simulink model "normalization"  (R2023b)
settings: Solver=VariableStepAuto  StartTime=0.0  StopTime=2  RelTol=1e-3
PreLoadFcn:
  | buffer_tiling
InitFcn:
  | buffer_tiling
values from neighbouring files (symbols this model uses):
  COL = 128    [run_model.m]
  inMat1 = reshape(inMat(1:ROW/PLIO_NUM,:)',[],1)    [run_model.m]
  inMat2 = reshape(inMat(ROW/PLIO_NUM+1:ROW/PLIO_NUM*2,:)',[],1)    [run_model.m]
  inMat3 = reshape(inMat(ROW/PLIO_NUM*2+1:ROW,:)',[],1)    [run_model.m]
  ROW = 384    [run_model.m]
undefined symbols (not defined in the file or in its folder): AIE, aie, es1, mean_dev_norm_first, mean_dev_norm_last, mean_dev_norm_middle, ML, mtxA_r, mtxA_w, mtxB_r, mtxB_w, S, vsvh1760, xcve2802
libraries: aieUtilities x14, aieBasic x14, vmcUtilities x1
settings Model: Creator=robg  LastModifiedBy=abehbood
settings DataIOCC: ReturnWorkspaceOutputs=off
settings OptimizationCC: ReuseModelBlockBuffer=off

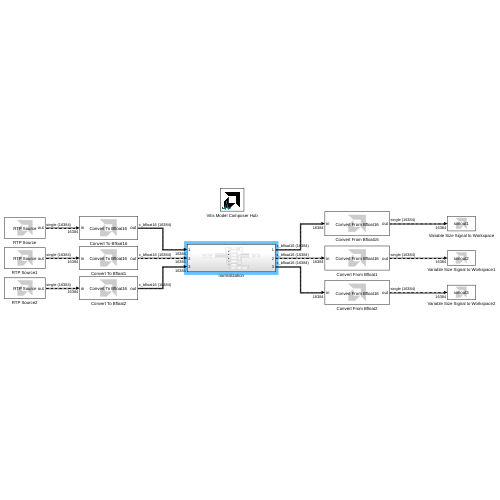
[thumbnail: Simulink's stored preview of the top-level diagram]
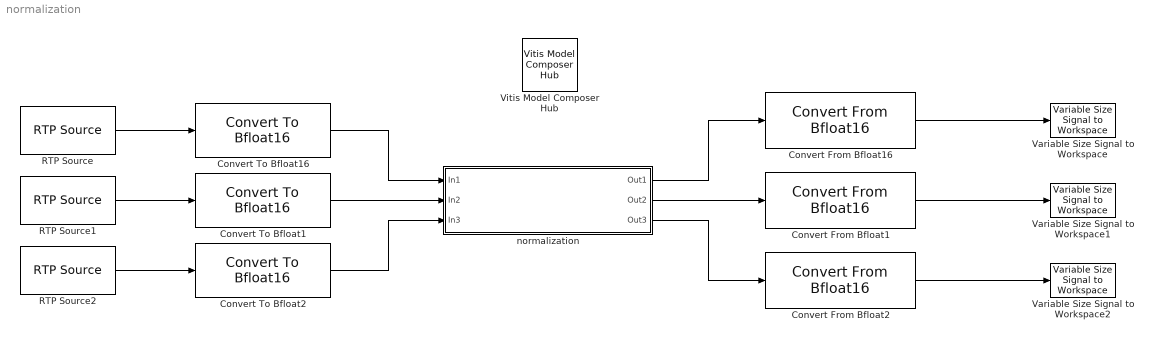
== system normalization ==
  Convert From Bfloat1 : aieUtilities/Convert From Bfloat16  OutputDataType=single
  Convert From Bfloat16 : aieUtilities/Convert From Bfloat16  OutputDataType=single
  Convert From Bfloat2 : aieUtilities/Convert From Bfloat16  OutputDataType=single
  Convert To Bfloat1 : aieUtilities/Convert To Bfloat16
  Convert To Bfloat16 : aieUtilities/Convert To Bfloat16
  Convert To Bfloat2 : aieUtilities/Convert To Bfloat16
  RTP Source : aieUtilities/RTP Source  Value=inMat1  SampleTime=1  OutputForm=Empty
  RTP Source1 : aieUtilities/RTP Source  Value=inMat2  SampleTime=1  OutputForm=Empty
  RTP Source2 : aieUtilities/RTP Source  Value=inMat3  SampleTime=1  OutputForm=Empty
  Variable Size Signal to Workspace : aieUtilities/Variable Size Signal to Workspace  VariableNameMask=simout1
  Variable Size Signal to Workspace1 : aieUtilities/Variable Size Signal to Workspace  VariableNameMask=simout2
  Variable Size Signal to Workspace2 : aieUtilities/Variable Size Signal to Workspace  VariableNameMask=simout3
  Vitis Model Composer Hub : vmcUtilities/Vitis Model Composer Hub  Tag=genX  CodeGeneration=off  SubsystemName=test  CompilationType=AIECompilation  ExportTypeV2=Graph Code  TargetDirectory=./code  exportDesign=off  analyzeDesign=on  validateDesignOnHw=off  ExportType=AI Engines  IpVendor=xilinx.com  IpLibrary=hls  IpVersion=1.0  IpHWLanguage=Verilog  AieCompilerOptions={}  AieSimulatorOptions={}  CreateTestbench=on  TestbenchStackSize=10  RunRtlSim=off  RunCSim=off  RunAieSim=on  AieSimTimeout=50000  RunAieSimProfiling=off  LaunchVitisAnalyzer=off  PlotOutput=off  RunX86Sim=off  X86SimTimeout=10  GenHwImage=off  GenLibadfXo=off  GenHwValidationCode=off  PlatformType=Specify Platform  Platform=/proj/xbuilds/SWIP/9999.0_0214_2115/installs/lin64/Vitis/2024.1/base_platforms/xilinx_vek280_es1_base_202410_1/xilinx_vek280_es1_base_202410_1.xpfm  HwSystemType=Baremetal  HwValidationTarget=hw  ProjDevice=Versal VEK280 ES1 Evaluation Platform with FMC Connector (xcve2802-vsvh1760-2MP-e-S-es1)  ProjDevicePart=xcve2802-vsvh1760-2MP-e-S-es1  AIEType=AIE-ML  SamplePeriod=-1  ClockFrequency=200  DataPathParallelism=1  xilinxfamily=versalaiedgees1  part=xcve2802  speed=-2MP-e-S-es1  package=vsvh1760  directory=./netlist  testbench=off  incr_netlist=off  synthesis_tool=Vivado  clock_wrapper=Clock Enables  dbl_ovrd=According to Block Masks  dcm_input_clock_period=10  sysclk_period=10  simulink_period=1  eval_field=0  IPInfoJsonString="{\"AIESubsystem\":{\"SubsystemName\":\"test\",\"TargetDirectory\":\"./code\",\"SubsystemDir\":\"./code/ip/test\"},\"SubsystemTag\":\"AIENode\"}"  LogFileName=/proj/xsjhdstaff4/abehbood/customers/AIE-ML_Performance_Analysis/normalization_v4/code/model_composer.log  NThreads=4
  normalization : Subsystem
  wires:
  RTP Source/1 -> Convert To Bfloat16/1
  Convert To Bfloat16/1 -> normalization/1(In1)
  normalization/1(Out1) -> Convert From Bfloat16/1
  Convert To Bfloat1/1 -> normalization/2(In2)
  RTP Source1/1 -> Convert To Bfloat1/1
  Convert To Bfloat2/1 -> normalization/3(In3)
  RTP Source2/1 -> Convert To Bfloat2/1
  normalization/2(Out2) -> Convert From Bfloat1/1
  normalization/3(Out3) -> Convert From Bfloat2/1
  Convert From Bfloat16/1 -> Variable Size Signal to Workspace/1
  Convert From Bfloat1/1 -> Variable Size Signal to Workspace1/1
  Convert From Bfloat2/1 -> Variable Size Signal to Workspace2/1

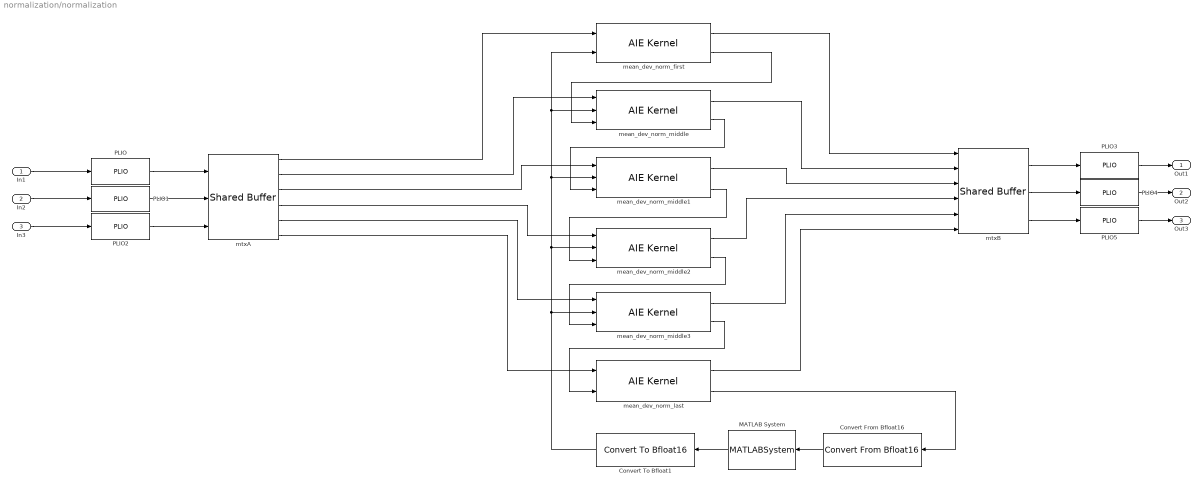
== system normalization/normalization ==
  In1 : Inport
  In2 : Inport  Port=2
  In3 : Inport  Port=3
  Convert From Bfloat16 : aieUtilities/Convert From Bfloat16  OutputDataType=single
  Convert To Bfloat1 : aieUtilities/Convert To Bfloat16
  MATLAB System : MATLABSystem  System=cycleBreaker  SimulateUsing=Interpreted execution
      mask Type: cycleBreaker
      mask Display:
      | disp('cycleBreaker');
      | port_label('input',1,'u');
      | port_label('output',1,'y');
  PLIO{,1..5} (6 alike) : aieBasic/PLIO  PlioWidth=128  PlioFreqSpec=off  PlioFreq=250  ColLocation=0  channel=0  blockJsonConstraints=[]  deprecateConstraints=0
  mean_dev_norm_first : aieBasic/AIE Kernel  KernelAllAttrs=|  PortNames={'data'; 'mean_dev'; 'out'; 'partial_out'}  PortSerializedTypes={'{Q2{R{Tadf::input_buffer{1{t{Sbfloat16}}}}}}'; '{Q2{P{Tinput_stream{1{t{Sbfloat16}}}}}}'; '{Q2{R{Tadf::output_buffer{1{t{Sbfloat16}}}}}}'; '{Q2{P{Toutput_cascade{2{t{Saccfloat}}{t{Bv}}}}}}'}  PortWindowSizes={8.192000000000000000e+03, 0.000000000000000000e+00, 8.192000000000000000e+03, 0.000000000000000000e+00}  PortWindowMargins={0.000000000000000000e+00, 0.000000000000000000e+00, 0.000000000000000000e+00, 0.000000000000000000e+00}  PortSynchronicities={'sync', 'auto', 'sync', 'auto'}  PortSignalSizes={0.000000000000000000e+00; 0.000000000000000000e+00; 0.000000000000000000e+00; 3.200000000000000000e+01}  FunctionTemplateSpecKind=implicit  FunctionTemplateParamNames={'COL'; 'ROW'}  FunctionTemplateParamKinds={'nontype'; 'nontype'}  FunctionTemplateParamTypes={'int'; 'int'}  FunctionTemplateParamValues={'128', '64'}  FunctionIndex=1  FunctionTabVisible=on  FunctionTemplateParamsVisible=on  FunctionDeclTypeOptions=|  FunctionDecl=|  FunctionTemplateParams={ 'COL', 'int', 'K_COL'; 'ROW', 'int', 'K_ROW' }  FunctionTemplateParamsEnables={'off', 'off', 'on';'off', 'off', 'on'}  PortAttrs={ 'input', 'data', 'adf::input_buffer< bfloat16 > & restrict', 'K_COL*K_ROW', '0', 'sync', ''; 'input', 'mean_dev', 'input_stream< bfloat16 > * restrict', '', '', '', ''; 'output', 'out', 'adf::output_buffer< bfloat16 > & restrict', 'K_COL*K_ROW', '', 'sync', ''; 'output', 'partial_out', 'output_cascade< accfloat, void > * restrict', '', '', '', '32' }  PortAttrsEnables={'off', 'off', 'off', 'on', 'off', 'off', 'off';'off', 'off', 'off', 'off', 'off', 'off', 'off';'off', 'off', 'off', 'on', 'off', 'off', 'off';'off', 'off', 'off', 'off', 'off', 'off', 'on'}  SampleTime=-1  KernelHeaderFile=aie/kernels.h  KernelFunction=mean_dev_norm_first  KernelSourceFile=aie/mean_dev_norm_first.cc  KernelSearchPaths={}  PreProcOptions={}  blockJsonConstraints=[]
      KernelAllAttrs=|
      | s[12;12;9;9;19;14;21;23;21;23;24;21;15;17;12;24;26;26;26;27;28;9;21;23;23;23;24;25;14;19;19;29]@FunctionNameDeclFileNamePortNamesPortTypesPortSerializedTypesPortDirectionsPortWindowSizeEnablesPortWindowMarginEnablesPortBufferSizeEnablesPortBufferMarginEnablesPortSynchronicityEnablesPortSignalSizeEnablesPortBufferSizesPortBufferMarginsFunctionDeclFunctionTemplateSpecKindFunctionTemplateParamNamesFunctionTemplateParamKindsFunctionTemplateParamTypesFunctionTemplateParamValuesFunctionTemplateParamEnablesClassDeclClassTemplateSpecKindClassTemplateParamNamesClassTemplateParamKindsClassTemplateParamTypesClassTemplateParamValuesClassTemplateParamEnablesClassCtorDeclsClassCtorParamNamesClassCtorParamTypesClassCtorParamSerializedTypes[1 1]@C[32 1]@t19@mean_dev_norm_firstt19@../../aie/kernels.hC[4 1]@t4@datat8@mean_devt3@outt11@partial_outC[4 1]@t40@adf::input_buffer< bfloat16 > & restrictt35@input_stream< bfloat16 > * restrictt41@adf::output_buffer< bfloat16 > & restrictt43@output_cascade< accfloat, void > * restrictC[4 1]@t44@{Q2{R{Tadf::input_buffer{1{t{Sbfloat16}}}}}}t39@{Q2{P{Tinput_stream{1{t{Sbfloat16}}}}}}t45@{Q2{R{Tadf::output_buffer{1{t{Sbfloat16}}}}}}t48@{Q2{P{Toutput_cascade{2{t{Saccfloat}}{t{Bv}}}}}}C[4 1]@t5@inputt5@inputt6@outputt6@outputC[4 1]@l1@l0@l1@l0@C[4 1]@l1@l0@l0@l0@C[4 1]@l1@l0@l1@l0@C[4 1]@l0@l0@l0@l0@C[4 1]@l1@l0@l1@l0@C[4 1]@l0@l0@l0@l1@C[4 1]@nnnnC[4 1]@nnnnt252@template < int COL, int ROW > 
      | void mean_dev_norm_first(adf::input_buffer< bfloat16 > & restrict data, input_stream< bfloat16 > * restrict mean_dev, adf::output_buffer< bfloat16 > & restrict out, output_cascade< accfloat, void > * restrict partial_out)t8@implicitC[2 1]@t3@COLt3@ROWC[2 1]@t7@nontypet7@nontypeC[2 1]@t3@intt3@intC[2 1]@nnC[2 1]@l1@l1@nne[0 1]@e[0 1]@e[0 1]@e[0 1]@e[0 1]@e[0 1]@e[0 1]@e[0 1]@e[0 1]@
      FunctionDeclTypeOptions=|
      | C[1 1]@t254@template < int COL, int ROW > 
      | void mean_dev_norm_first(adf::input_buffer< bfloat16 > && restrict data, input_stream< bfloat16 > * restrict mean_dev, adf::output_buffer< bfloat16 > && restrict out, output_cascade< accfloat, void > * restrict partial_out)
      FunctionDecl=|
      | template < int COL, int ROW > 
      | void mean_dev_norm_first(adf::input_buffer< bfloat16 > && restrict data, input_stream< bfloat16 > * restrict mean_dev, adf::output_buffer< bfloat16 > && restrict out, output_cascade< accfloat, void > * restrict partial_out)
  mean_dev_norm_last : aieBasic/AIE Kernel  KernelAllAttrs=|  PortNames={'data'; 'partial_in'; 'out'; 'mean_dev_out'}  PortSerializedTypes={'{Q2{R{Tadf::input_buffer{1{t{Sbfloat16}}}}}}'; '{Q2{P{Tinput_cascade{2{t{Saccfloat}}{t{Bv}}}}}}'; '{Q2{R{Tadf::output_buffer{1{t{Sbfloat16}}}}}}'; '{Q2{P{Toutput_stream{1{t{Sbfloat16}}}}}}'}  PortWindowSizes={8.192000000000000000e+03, 0.000000000000000000e+00, 8.192000000000000000e+03, 0.000000000000000000e+00}  PortWindowMargins={0.000000000000000000e+00, 0.000000000000000000e+00, 0.000000000000000000e+00, 0.000000000000000000e+00}  PortSynchronicities={'sync', 'auto', 'sync', 'auto'}  PortSignalSizes={0.000000000000000000e+00; 0.000000000000000000e+00; 0.000000000000000000e+00; 2.000000000000000000e+00}  FunctionTemplateSpecKind=implicit  FunctionTemplateParamNames={'COL'; 'ROW'; 'NUM'}  FunctionTemplateParamKinds={'nontype'; 'nontype'; 'nontype'}  FunctionTemplateParamTypes={'int'; 'int'; 'int'}  FunctionTemplateParamValues={'128', '64', '6'}  FunctionIndex=1  FunctionTabVisible=on  FunctionTemplateParamsVisible=on  FunctionDeclTypeOptions=|  FunctionDecl=|  FunctionTemplateParams={ 'COL', 'int', 'K_COL'; 'ROW', 'int', 'K_ROW'; 'NUM', 'int', 'NUM' }  FunctionTemplateParamsEnables={'off', 'off', 'on';'off', 'off', 'on';'off', 'off', 'on'}  PortAttrs={ 'input', 'data', 'adf::input_buffer< bfloat16 > & restrict', 'K_COL*K_ROW', '0', 'sync', ''; 'input', 'partial_in', 'input_cascade< accfloat, void > * restrict', '', '', '', ''; 'output', 'out', 'adf::output_buffer< bfloat16 > & restrict', 'K_COL*K_ROW', '', 'sync', ''; 'output', 'mean_dev_out', 'output_stream< bfloat16 > * restrict', '', '', '', '2' }  PortAttrsEnables={'off', 'off', 'off', 'on', 'off', 'off', 'off';'off', 'off', 'off', 'off', 'off', 'off', 'off';'off', 'off', 'off', 'on', 'off', 'off', 'off';'off', 'off', 'off', 'off', 'off', 'off', 'on'}  SampleTime=-1  KernelHeaderFile=aie/kernels.h  KernelFunction=mean_dev_norm_last  KernelSourceFile=aie/mean_dev_norm_last.cc  KernelSearchPaths={}  PreProcOptions={}  blockJsonConstraints=[]
      KernelAllAttrs=|
      | s[12;12;9;9;19;14;21;23;21;23;24;21;15;17;12;24;26;26;26;27;28;9;21;23;23;23;24;25;14;19;19;29]@FunctionNameDeclFileNamePortNamesPortTypesPortSerializedTypesPortDirectionsPortWindowSizeEnablesPortWindowMarginEnablesPortBufferSizeEnablesPortBufferMarginEnablesPortSynchronicityEnablesPortSignalSizeEnablesPortBufferSizesPortBufferMarginsFunctionDeclFunctionTemplateSpecKindFunctionTemplateParamNamesFunctionTemplateParamKindsFunctionTemplateParamTypesFunctionTemplateParamValuesFunctionTemplateParamEnablesClassDeclClassTemplateSpecKindClassTemplateParamNamesClassTemplateParamKindsClassTemplateParamTypesClassTemplateParamValuesClassTemplateParamEnablesClassCtorDeclsClassCtorParamNamesClassCtorParamTypesClassCtorParamSerializedTypes[1 1]@C[32 1]@t18@mean_dev_norm_lastt19@../../aie/kernels.hC[4 1]@t4@datat10@partial_int3@outt12@mean_dev_outC[4 1]@t40@adf::input_buffer< bfloat16 > & restrictt42@input_cascade< accfloat, void > * restrictt41@adf::output_buffer< bfloat16 > & restrictt36@output_stream< bfloat16 > * restrictC[4 1]@t44@{Q2{R{Tadf::input_buffer{1{t{Sbfloat16}}}}}}t47@{Q2{P{Tinput_cascade{2{t{Saccfloat}}{t{Bv}}}}}}t45@{Q2{R{Tadf::output_buffer{1{t{Sbfloat16}}}}}}t40@{Q2{P{Toutput_stream{1{t{Sbfloat16}}}}}}C[4 1]@t5@inputt5@inputt6@outputt6@outputC[4 1]@l1@l0@l1@l0@C[4 1]@l1@l0@l0@l0@C[4 1]@l1@l0@l1@l0@C[4 1]@l0@l0@l0@l0@C[4 1]@l1@l0@l1@l0@C[4 1]@l0@l0@l0@l1@C[4 1]@nnnnC[4 1]@nnnnt263@template < int COL, int ROW, int NUM > 
      | void mean_dev_norm_last(adf::input_buffer< bfloat16 > & restrict data, input_cascade< accfloat, void > * restrict partial_in, adf::output_buffer< bfloat16 > & restrict out, output_stream< bfloat16 > * restrict mean_dev_out)t8@implicitC[3 1]@t3@COLt3@ROWt3@NUMC[3 1]@t7@nontypet7@nontypet7@nontypeC[3 1]@t3@intt3@intt3@intC[3 1]@nnnC[3 1]@l1@l1@l1@nne[0 1]@e[0 1]@e[0 1]@e[0 1]@e[0 1]@e[0 1]@e[0 1]@e[0 1]@e[0 1]@
      FunctionDeclTypeOptions=|
      | C[1 1]@t265@template < int COL, int ROW, int NUM > 
      | void mean_dev_norm_last(adf::input_buffer< bfloat16 > && restrict data, input_cascade< accfloat, void > * restrict partial_in, adf::output_buffer< bfloat16 > && restrict out, output_stream< bfloat16 > * restrict mean_dev_out)
      FunctionDecl=|
      | template < int COL, int ROW, int NUM > 
      | void mean_dev_norm_last(adf::input_buffer< bfloat16 > && restrict data, input_cascade< accfloat, void > * restrict partial_in, adf::output_buffer< bfloat16 > && restrict out, output_stream< bfloat16 > * restrict mean_dev_out)
  mean_dev_norm_middle : aieBasic/AIE Kernel  KernelAllAttrs=|  PortNames={'data'; 'mean_dev'; 'partial_in'; 'out'; 'partial_out'}  PortSerializedTypes={'{Q2{R{Tadf::input_buffer{1{t{Sbfloat16}}}}}}'; '{Q2{P{Tinput_stream{1{t{Sbfloat16}}}}}}'; '{Q2{P{Tinput_cascade{2{t{Saccfloat}}{t{Bv}}}}}}'; '{Q2{R{Tadf::output_buffer{1{t{Sbfloat16}}}}}}'; '{Q2{P{Toutput_cascade{2{t{Saccfloat}}{t{Bv}}}}}}'}  PortWindowSizes={8.192000000000000000e+03, 0.000000000000000000e+00, 0.000000000000000000e+00, 8.192000000000000000e+03, 0.000000000000000000e+00}  PortWindowMargins={0.000000000000000000e+00, 0.000000000000000000e+00, 0.000000000000000000e+00, 0.000000000000000000e+00, 0.000000000000000000e+00}  PortSynchronicities={'sync', 'auto', 'auto', 'sync', 'auto'}  PortSignalSizes={0.000000000000000000e+00; 0.000000000000000000e+00; 0.000000000000000000e+00; 0.000000000000000000e+00; 3.200000000000000000e+01}  FunctionTemplateSpecKind=implicit  FunctionTemplateParamNames={'COL'; 'ROW'}  FunctionTemplateParamKinds={'nontype'; 'nontype'}  FunctionTemplateParamTypes={'int'; 'int'}  FunctionTemplateParamValues={'128', '64'}  FunctionIndex=1  FunctionTabVisible=on  FunctionTemplateParamsVisible=on  FunctionDeclTypeOptions=|  FunctionDecl=|  FunctionTemplateParams={ 'COL', 'int', 'K_COL'; 'ROW', 'int', 'K_ROW' }  FunctionTemplateParamsEnables={'off', 'off', 'on';'off', 'off', 'on'}  PortAttrs={ 'input', 'data', 'adf::input_buffer< bfloat16 > & restrict', 'K_COL*K_ROW', '0', 'sync', ''; 'input', 'mean_dev', 'input_stream< bfloat16 > * restrict', '', '', '', ''; 'input', 'partial_in', 'input_cascade< accfloat, void > * restrict', '', '', '', ''; 'output', 'out', 'adf::output_buffer< bfloat16 > & restrict', 'K_COL*K_ROW', '', 'sync', ''; 'output', 'partial_out', 'output_cascade< accfloat, void > * restrict', '', '', '', '32' }  PortAttrsEnables={'off', 'off', 'off', 'on', 'off', 'off', 'off';'off', 'off', 'off', 'off', 'off', 'off', 'off';'off', 'off', 'off', 'off', 'off', 'off', 'off';'off', 'off', 'off', 'on', 'off', 'off', 'off';'off', 'off', 'off', 'off', 'off', 'off', 'on'}  SampleTime=-1  KernelHeaderFile=aie/kernels.h  KernelFunction=mean_dev_norm_middle  KernelSourceFile=aie/mean_dev_norm_middle.cc  KernelSearchPaths={}  PreProcOptions={}  blockJsonConstraints=[]
      KernelAllAttrs=|
      | s[12;12;9;9;19;14;21;23;21;23;24;21;15;17;12;24;26;26;26;27;28;9;21;23;23;23;24;25;14;19;19;29]@FunctionNameDeclFileNamePortNamesPortTypesPortSerializedTypesPortDirectionsPortWindowSizeEnablesPortWindowMarginEnablesPortBufferSizeEnablesPortBufferMarginEnablesPortSynchronicityEnablesPortSignalSizeEnablesPortBufferSizesPortBufferMarginsFunctionDeclFunctionTemplateSpecKindFunctionTemplateParamNamesFunctionTemplateParamKindsFunctionTemplateParamTypesFunctionTemplateParamValuesFunctionTemplateParamEnablesClassDeclClassTemplateSpecKindClassTemplateParamNamesClassTemplateParamKindsClassTemplateParamTypesClassTemplateParamValuesClassTemplateParamEnablesClassCtorDeclsClassCtorParamNamesClassCtorParamTypesClassCtorParamSerializedTypes[1 1]@C[32 1]@t20@mean_dev_norm_middlet19@../../aie/kernels.hC[5 1]@t4@datat8@mean_devt10@partial_int3@outt11@partial_outC[5 1]@t40@adf::input_buffer< bfloat16 > & restrictt35@input_stream< bfloat16 > * restrictt42@input_cascade< accfloat, void > * restrictt41@adf::output_buffer< bfloat16 > & restrictt43@output_cascade< accfloat, void > * restrictC[5 1]@t44@{Q2{R{Tadf::input_buffer{1{t{Sbfloat16}}}}}}t39@{Q2{P{Tinput_stream{1{t{Sbfloat16}}}}}}t47@{Q2{P{Tinput_cascade{2{t{Saccfloat}}{t{Bv}}}}}}t45@{Q2{R{Tadf::output_buffer{1{t{Sbfloat16}}}}}}t48@{Q2{P{Toutput_cascade{2{t{Saccfloat}}{t{Bv}}}}}}C[5 1]@t5@inputt5@inputt5@inputt6@outputt6@outputC[5 1]@l1@l0@l0@l1@l0@C[5 1]@l1@l0@l0@l0@l0@C[5 1]@l1@l0@l0@l1@l0@C[5 1]@l0@l0@l0@l0@l0@C[5 1]@l1@l0@l0@l1@l0@C[5 1]@l0@l0@l0@l0@l1@C[5 1]@nnnnnC[5 1]@nnnnnt308@template < int COL, int ROW > 
      | void mean_dev_norm_middle(adf::input_buffer< bfloat16 > & restrict data, input_stream< bfloat16 > * restrict mean_dev, input_cascade< accfloat, void > * restrict partial_in, adf::output_buffer< bfloat16 > & restrict out, output_cascade< accfloat, void > * restrict partial_out)t8@implicitC[2 1]@t3@COLt3@ROWC[2 1]@t7@nontypet7@nontypeC[2 1]@t3@intt3@intC[2 1]@nnC[2 1]@l1@l1@nne[0 1]@e[0 1]@e[0 1]@e[0 1]@e[0 1]@e[0 1]@e[0 1]@e[0 1]@e[0 1]@
      FunctionDeclTypeOptions=|
      | C[1 1]@t310@template < int COL, int ROW > 
      | void mean_dev_norm_middle(adf::input_buffer< bfloat16 > && restrict data, input_stream< bfloat16 > * restrict mean_dev, input_cascade< accfloat, void > * restrict partial_in, adf::output_buffer< bfloat16 > && restrict out, output_cascade< accfloat, void > * restrict partial_out)
      FunctionDecl=|
      | template < int COL, int ROW > 
      | void mean_dev_norm_middle(adf::input_buffer< bfloat16 > && restrict data, input_stream< bfloat16 > * restrict mean_dev, input_cascade< accfloat, void > * restrict partial_in, adf::output_buffer< bfloat16 > && restrict out, output_cascade< accfloat, void > * restrict partial_out)
  mean_dev_norm_middle1 : aieBasic/AIE Kernel  KernelAllAttrs=|  PortNames={'data'; 'mean_dev'; 'partial_in'; 'out'; 'partial_out'}  PortSerializedTypes={'{Q2{R{Tadf::input_buffer{1{t{Sbfloat16}}}}}}'; '{Q2{P{Tinput_stream{1{t{Sbfloat16}}}}}}'; '{Q2{P{Tinput_cascade{2{t{Saccfloat}}{t{Bv}}}}}}'; '{Q2{R{Tadf::output_buffer{1{t{Sbfloat16}}}}}}'; '{Q2{P{Toutput_cascade{2{t{Saccfloat}}{t{Bv}}}}}}'}  PortWindowSizes={8.192000000000000000e+03, 0.000000000000000000e+00, 0.000000000000000000e+00, 8.192000000000000000e+03, 0.000000000000000000e+00}  PortWindowMargins={0.000000000000000000e+00, 0.000000000000000000e+00, 0.000000000000000000e+00, 0.000000000000000000e+00, 0.000000000000000000e+00}  PortSynchronicities={'sync', 'auto', 'auto', 'sync', 'auto'}  PortSignalSizes={0.000000000000000000e+00; 0.000000000000000000e+00; 0.000000000000000000e+00; 0.000000000000000000e+00; 3.200000000000000000e+01}  FunctionTemplateSpecKind=implicit  FunctionTemplateParamNames={'COL'; 'ROW'}  FunctionTemplateParamKinds={'nontype'; 'nontype'}  FunctionTemplateParamTypes={'int'; 'int'}  FunctionTemplateParamValues={'128', '64'}  FunctionIndex=1  FunctionTabVisible=on  FunctionTemplateParamsVisible=on  FunctionDeclTypeOptions=|  FunctionDecl=|  FunctionTemplateParams={ 'COL', 'int', 'K_COL'; 'ROW', 'int', 'K_ROW' }  FunctionTemplateParamsEnables={'off', 'off', 'on';'off', 'off', 'on'}  PortAttrs={ 'input', 'data', 'adf::input_buffer< bfloat16 > & restrict', 'K_COL*K_ROW', '0', 'sync', ''; 'input', 'mean_dev', 'input_stream< bfloat16 > * restrict', '', '', '', ''; 'input', 'partial_in', 'input_cascade< accfloat, void > * restrict', '', '', '', ''; 'output', 'out', 'adf::output_buffer< bfloat16 > & restrict', 'K_COL*K_ROW', '', 'sync', ''; 'output', 'partial_out', 'output_cascade< accfloat, void > * restrict', '', '', '', '32' }  PortAttrsEnables={'off', 'off', 'off', 'on', 'off', 'off', 'off';'off', 'off', 'off', 'off', 'off', 'off', 'off';'off', 'off', 'off', 'off', 'off', 'off', 'off';'off', 'off', 'off', 'on', 'off', 'off', 'off';'off', 'off', 'off', 'off', 'off', 'off', 'on'}  SampleTime=-1  KernelHeaderFile=aie/kernels.h  KernelFunction=mean_dev_norm_middle  KernelSourceFile=aie/mean_dev_norm_middle.cc  KernelSearchPaths={}  PreProcOptions={}  blockJsonConstraints=[]
      KernelAllAttrs=|
      | s[12;12;9;9;19;14;21;23;21;23;24;21;15;17;12;24;26;26;26;27;28;9;21;23;23;23;24;25;14;19;19;29]@FunctionNameDeclFileNamePortNamesPortTypesPortSerializedTypesPortDirectionsPortWindowSizeEnablesPortWindowMarginEnablesPortBufferSizeEnablesPortBufferMarginEnablesPortSynchronicityEnablesPortSignalSizeEnablesPortBufferSizesPortBufferMarginsFunctionDeclFunctionTemplateSpecKindFunctionTemplateParamNamesFunctionTemplateParamKindsFunctionTemplateParamTypesFunctionTemplateParamValuesFunctionTemplateParamEnablesClassDeclClassTemplateSpecKindClassTemplateParamNamesClassTemplateParamKindsClassTemplateParamTypesClassTemplateParamValuesClassTemplateParamEnablesClassCtorDeclsClassCtorParamNamesClassCtorParamTypesClassCtorParamSerializedTypes[1 1]@C[32 1]@t20@mean_dev_norm_middlet19@../../aie/kernels.hC[5 1]@t4@datat8@mean_devt10@partial_int3@outt11@partial_outC[5 1]@t40@adf::input_buffer< bfloat16 > & restrictt35@input_stream< bfloat16 > * restrictt42@input_cascade< accfloat, void > * restrictt41@adf::output_buffer< bfloat16 > & restrictt43@output_cascade< accfloat, void > * restrictC[5 1]@t44@{Q2{R{Tadf::input_buffer{1{t{Sbfloat16}}}}}}t39@{Q2{P{Tinput_stream{1{t{Sbfloat16}}}}}}t47@{Q2{P{Tinput_cascade{2{t{Saccfloat}}{t{Bv}}}}}}t45@{Q2{R{Tadf::output_buffer{1{t{Sbfloat16}}}}}}t48@{Q2{P{Toutput_cascade{2{t{Saccfloat}}{t{Bv}}}}}}C[5 1]@t5@inputt5@inputt5@inputt6@outputt6@outputC[5 1]@l1@l0@l0@l1@l0@C[5 1]@l1@l0@l0@l0@l0@C[5 1]@l1@l0@l0@l1@l0@C[5 1]@l0@l0@l0@l0@l0@C[5 1]@l1@l0@l0@l1@l0@C[5 1]@l0@l0@l0@l0@l1@C[5 1]@nnnnnC[5 1]@nnnnnt308@template < int COL, int ROW > 
      | void mean_dev_norm_middle(adf::input_buffer< bfloat16 > & restrict data, input_stream< bfloat16 > * restrict mean_dev, input_cascade< accfloat, void > * restrict partial_in, adf::output_buffer< bfloat16 > & restrict out, output_cascade< accfloat, void > * restrict partial_out)t8@implicitC[2 1]@t3@COLt3@ROWC[2 1]@t7@nontypet7@nontypeC[2 1]@t3@intt3@intC[2 1]@nnC[2 1]@l1@l1@nne[0 1]@e[0 1]@e[0 1]@e[0 1]@e[0 1]@e[0 1]@e[0 1]@e[0 1]@e[0 1]@
      FunctionDeclTypeOptions=|
      | C[1 1]@t310@template < int COL, int ROW > 
      | void mean_dev_norm_middle(adf::input_buffer< bfloat16 > && restrict data, input_stream< bfloat16 > * restrict mean_dev, input_cascade< accfloat, void > * restrict partial_in, adf::output_buffer< bfloat16 > && restrict out, output_cascade< accfloat, void > * restrict partial_out)
      FunctionDecl=|
      | template < int COL, int ROW > 
      | void mean_dev_norm_middle(adf::input_buffer< bfloat16 > && restrict data, input_stream< bfloat16 > * restrict mean_dev, input_cascade< accfloat, void > * restrict partial_in, adf::output_buffer< bfloat16 > && restrict out, output_cascade< accfloat, void > * restrict partial_out)
  mean_dev_norm_middle2 : aieBasic/AIE Kernel  KernelAllAttrs=|  PortNames={'data'; 'mean_dev'; 'partial_in'; 'out'; 'partial_out'}  PortSerializedTypes={'{Q2{R{Tadf::input_buffer{1{t{Sbfloat16}}}}}}'; '{Q2{P{Tinput_stream{1{t{Sbfloat16}}}}}}'; '{Q2{P{Tinput_cascade{2{t{Saccfloat}}{t{Bv}}}}}}'; '{Q2{R{Tadf::output_buffer{1{t{Sbfloat16}}}}}}'; '{Q2{P{Toutput_cascade{2{t{Saccfloat}}{t{Bv}}}}}}'}  PortWindowSizes={8.192000000000000000e+03, 0.000000000000000000e+00, 0.000000000000000000e+00, 8.192000000000000000e+03, 0.000000000000000000e+00}  PortWindowMargins={0.000000000000000000e+00, 0.000000000000000000e+00, 0.000000000000000000e+00, 0.000000000000000000e+00, 0.000000000000000000e+00}  PortSynchronicities={'sync', 'auto', 'auto', 'sync', 'auto'}  PortSignalSizes={0.000000000000000000e+00; 0.000000000000000000e+00; 0.000000000000000000e+00; 0.000000000000000000e+00; 3.200000000000000000e+01}  FunctionTemplateSpecKind=implicit  FunctionTemplateParamNames={'COL'; 'ROW'}  FunctionTemplateParamKinds={'nontype'; 'nontype'}  FunctionTemplateParamTypes={'int'; 'int'}  FunctionTemplateParamValues={'128', '64'}  FunctionIndex=1  FunctionTabVisible=on  FunctionTemplateParamsVisible=on  FunctionDeclTypeOptions=|  FunctionDecl=|  FunctionTemplateParams={ 'COL', 'int', 'K_COL'; 'ROW', 'int', 'K_ROW' }  FunctionTemplateParamsEnables={'off', 'off', 'on';'off', 'off', 'on'}  PortAttrs={ 'input', 'data', 'adf::input_buffer< bfloat16 > & restrict', 'K_COL*K_ROW', '0', 'sync', ''; 'input', 'mean_dev', 'input_stream< bfloat16 > * restrict', '', '', '', ''; 'input', 'partial_in', 'input_cascade< accfloat, void > * restrict', '', '', '', ''; 'output', 'out', 'adf::output_buffer< bfloat16 > & restrict', 'K_COL*K_ROW', '', 'sync', ''; 'output', 'partial_out', 'output_cascade< accfloat, void > * restrict', '', '', '', '32' }  PortAttrsEnables={'off', 'off', 'off', 'on', 'off', 'off', 'off';'off', 'off', 'off', 'off', 'off', 'off', 'off';'off', 'off', 'off', 'off', 'off', 'off', 'off';'off', 'off', 'off', 'on', 'off', 'off', 'off';'off', 'off', 'off', 'off', 'off', 'off', 'on'}  SampleTime=-1  KernelHeaderFile=aie/kernels.h  KernelFunction=mean_dev_norm_middle  KernelSourceFile=aie/mean_dev_norm_middle.cc  KernelSearchPaths={}  PreProcOptions={}  blockJsonConstraints=[]
      KernelAllAttrs=|
      | s[12;12;9;9;19;14;21;23;21;23;24;21;15;17;12;24;26;26;26;27;28;9;21;23;23;23;24;25;14;19;19;29]@FunctionNameDeclFileNamePortNamesPortTypesPortSerializedTypesPortDirectionsPortWindowSizeEnablesPortWindowMarginEnablesPortBufferSizeEnablesPortBufferMarginEnablesPortSynchronicityEnablesPortSignalSizeEnablesPortBufferSizesPortBufferMarginsFunctionDeclFunctionTemplateSpecKindFunctionTemplateParamNamesFunctionTemplateParamKindsFunctionTemplateParamTypesFunctionTemplateParamValuesFunctionTemplateParamEnablesClassDeclClassTemplateSpecKindClassTemplateParamNamesClassTemplateParamKindsClassTemplateParamTypesClassTemplateParamValuesClassTemplateParamEnablesClassCtorDeclsClassCtorParamNamesClassCtorParamTypesClassCtorParamSerializedTypes[1 1]@C[32 1]@t20@mean_dev_norm_middlet19@../../aie/kernels.hC[5 1]@t4@datat8@mean_devt10@partial_int3@outt11@partial_outC[5 1]@t40@adf::input_buffer< bfloat16 > & restrictt35@input_stream< bfloat16 > * restrictt42@input_cascade< accfloat, void > * restrictt41@adf::output_buffer< bfloat16 > & restrictt43@output_cascade< accfloat, void > * restrictC[5 1]@t44@{Q2{R{Tadf::input_buffer{1{t{Sbfloat16}}}}}}t39@{Q2{P{Tinput_stream{1{t{Sbfloat16}}}}}}t47@{Q2{P{Tinput_cascade{2{t{Saccfloat}}{t{Bv}}}}}}t45@{Q2{R{Tadf::output_buffer{1{t{Sbfloat16}}}}}}t48@{Q2{P{Toutput_cascade{2{t{Saccfloat}}{t{Bv}}}}}}C[5 1]@t5@inputt5@inputt5@inputt6@outputt6@outputC[5 1]@l1@l0@l0@l1@l0@C[5 1]@l1@l0@l0@l0@l0@C[5 1]@l1@l0@l0@l1@l0@C[5 1]@l0@l0@l0@l0@l0@C[5 1]@l1@l0@l0@l1@l0@C[5 1]@l0@l0@l0@l0@l1@C[5 1]@nnnnnC[5 1]@nnnnnt308@template < int COL, int ROW > 
      | void mean_dev_norm_middle(adf::input_buffer< bfloat16 > & restrict data, input_stream< bfloat16 > * restrict mean_dev, input_cascade< accfloat, void > * restrict partial_in, adf::output_buffer< bfloat16 > & restrict out, output_cascade< accfloat, void > * restrict partial_out)t8@implicitC[2 1]@t3@COLt3@ROWC[2 1]@t7@nontypet7@nontypeC[2 1]@t3@intt3@intC[2 1]@nnC[2 1]@l1@l1@nne[0 1]@e[0 1]@e[0 1]@e[0 1]@e[0 1]@e[0 1]@e[0 1]@e[0 1]@e[0 1]@
      FunctionDeclTypeOptions=|
      | C[1 1]@t310@template < int COL, int ROW > 
      | void mean_dev_norm_middle(adf::input_buffer< bfloat16 > && restrict data, input_stream< bfloat16 > * restrict mean_dev, input_cascade< accfloat, void > * restrict partial_in, adf::output_buffer< bfloat16 > && restrict out, output_cascade< accfloat, void > * restrict partial_out)
      FunctionDecl=|
      | template < int COL, int ROW > 
      | void mean_dev_norm_middle(adf::input_buffer< bfloat16 > && restrict data, input_stream< bfloat16 > * restrict mean_dev, input_cascade< accfloat, void > * restrict partial_in, adf::output_buffer< bfloat16 > && restrict out, output_cascade< accfloat, void > * restrict partial_out)
  mean_dev_norm_middle3 : aieBasic/AIE Kernel  KernelAllAttrs=|  PortNames={'data'; 'mean_dev'; 'partial_in'; 'out'; 'partial_out'}  PortSerializedTypes={'{Q2{R{Tadf::input_buffer{1{t{Sbfloat16}}}}}}'; '{Q2{P{Tinput_stream{1{t{Sbfloat16}}}}}}'; '{Q2{P{Tinput_cascade{2{t{Saccfloat}}{t{Bv}}}}}}'; '{Q2{R{Tadf::output_buffer{1{t{Sbfloat16}}}}}}'; '{Q2{P{Toutput_cascade{2{t{Saccfloat}}{t{Bv}}}}}}'}  PortWindowSizes={8.192000000000000000e+03, 0.000000000000000000e+00, 0.000000000000000000e+00, 8.192000000000000000e+03, 0.000000000000000000e+00}  PortWindowMargins={0.000000000000000000e+00, 0.000000000000000000e+00, 0.000000000000000000e+00, 0.000000000000000000e+00, 0.000000000000000000e+00}  PortSynchronicities={'sync', 'auto', 'auto', 'sync', 'auto'}  PortSignalSizes={0.000000000000000000e+00; 0.000000000000000000e+00; 0.000000000000000000e+00; 0.000000000000000000e+00; 3.200000000000000000e+01}  FunctionTemplateSpecKind=implicit  FunctionTemplateParamNames={'COL'; 'ROW'}  FunctionTemplateParamKinds={'nontype'; 'nontype'}  FunctionTemplateParamTypes={'int'; 'int'}  FunctionTemplateParamValues={'128', '64'}  FunctionIndex=1  FunctionTabVisible=on  FunctionTemplateParamsVisible=on  FunctionDeclTypeOptions=|  FunctionDecl=|  FunctionTemplateParams={ 'COL', 'int', 'K_COL'; 'ROW', 'int', 'K_ROW' }  FunctionTemplateParamsEnables={'off', 'off', 'on';'off', 'off', 'on'}  PortAttrs={ 'input', 'data', 'adf::input_buffer< bfloat16 > & restrict', 'K_COL*K_ROW', '0', 'sync', ''; 'input', 'mean_dev', 'input_stream< bfloat16 > * restrict', '', '', '', ''; 'input', 'partial_in', 'input_cascade< accfloat, void > * restrict', '', '', '', ''; 'output', 'out', 'adf::output_buffer< bfloat16 > & restrict', 'K_COL*K_ROW', '', 'sync', ''; 'output', 'partial_out', 'output_cascade< accfloat, void > * restrict', '', '', '', '32' }  PortAttrsEnables={'off', 'off', 'off', 'on', 'off', 'off', 'off';'off', 'off', 'off', 'off', 'off', 'off', 'off';'off', 'off', 'off', 'off', 'off', 'off', 'off';'off', 'off', 'off', 'on', 'off', 'off', 'off';'off', 'off', 'off', 'off', 'off', 'off', 'on'}  SampleTime=-1  KernelHeaderFile=aie/kernels.h  KernelFunction=mean_dev_norm_middle  KernelSourceFile=aie/mean_dev_norm_middle.cc  KernelSearchPaths={}  PreProcOptions={}  blockJsonConstraints=[]
      KernelAllAttrs=|
      | s[12;12;9;9;19;14;21;23;21;23;24;21;15;17;12;24;26;26;26;27;28;9;21;23;23;23;24;25;14;19;19;29]@FunctionNameDeclFileNamePortNamesPortTypesPortSerializedTypesPortDirectionsPortWindowSizeEnablesPortWindowMarginEnablesPortBufferSizeEnablesPortBufferMarginEnablesPortSynchronicityEnablesPortSignalSizeEnablesPortBufferSizesPortBufferMarginsFunctionDeclFunctionTemplateSpecKindFunctionTemplateParamNamesFunctionTemplateParamKindsFunctionTemplateParamTypesFunctionTemplateParamValuesFunctionTemplateParamEnablesClassDeclClassTemplateSpecKindClassTemplateParamNamesClassTemplateParamKindsClassTemplateParamTypesClassTemplateParamValuesClassTemplateParamEnablesClassCtorDeclsClassCtorParamNamesClassCtorParamTypesClassCtorParamSerializedTypes[1 1]@C[32 1]@t20@mean_dev_norm_middlet19@../../aie/kernels.hC[5 1]@t4@datat8@mean_devt10@partial_int3@outt11@partial_outC[5 1]@t40@adf::input_buffer< bfloat16 > & restrictt35@input_stream< bfloat16 > * restrictt42@input_cascade< accfloat, void > * restrictt41@adf::output_buffer< bfloat16 > & restrictt43@output_cascade< accfloat, void > * restrictC[5 1]@t44@{Q2{R{Tadf::input_buffer{1{t{Sbfloat16}}}}}}t39@{Q2{P{Tinput_stream{1{t{Sbfloat16}}}}}}t47@{Q2{P{Tinput_cascade{2{t{Saccfloat}}{t{Bv}}}}}}t45@{Q2{R{Tadf::output_buffer{1{t{Sbfloat16}}}}}}t48@{Q2{P{Toutput_cascade{2{t{Saccfloat}}{t{Bv}}}}}}C[5 1]@t5@inputt5@inputt5@inputt6@outputt6@outputC[5 1]@l1@l0@l0@l1@l0@C[5 1]@l1@l0@l0@l0@l0@C[5 1]@l1@l0@l0@l1@l0@C[5 1]@l0@l0@l0@l0@l0@C[5 1]@l1@l0@l0@l1@l0@C[5 1]@l0@l0@l0@l0@l1@C[5 1]@nnnnnC[5 1]@nnnnnt308@template < int COL, int ROW > 
      | void mean_dev_norm_middle(adf::input_buffer< bfloat16 > & restrict data, input_stream< bfloat16 > * restrict mean_dev, input_cascade< accfloat, void > * restrict partial_in, adf::output_buffer< bfloat16 > & restrict out, output_cascade< accfloat, void > * restrict partial_out)t8@implicitC[2 1]@t3@COLt3@ROWC[2 1]@t7@nontypet7@nontypeC[2 1]@t3@intt3@intC[2 1]@nnC[2 1]@l1@l1@nne[0 1]@e[0 1]@e[0 1]@e[0 1]@e[0 1]@e[0 1]@e[0 1]@e[0 1]@e[0 1]@
      FunctionDeclTypeOptions=|
      | C[1 1]@t310@template < int COL, int ROW > 
      | void mean_dev_norm_middle(adf::input_buffer< bfloat16 > && restrict data, input_stream< bfloat16 > * restrict mean_dev, input_cascade< accfloat, void > * restrict partial_in, adf::output_buffer< bfloat16 > && restrict out, output_cascade< accfloat, void > * restrict partial_out)
      FunctionDecl=|
      | template < int COL, int ROW > 
      | void mean_dev_norm_middle(adf::input_buffer< bfloat16 > && restrict data, input_stream< bfloat16 > * restrict mean_dev, input_cascade< accfloat, void > * restrict partial_in, adf::output_buffer< bfloat16 > && restrict out, output_cascade< accfloat, void > * restrict partial_out)
  mtxA : aieBasic/Shared Buffer  DataType=bfloat16  NumBuffer=1  BufferDim=[ROW,COL]  NumInput=3  NumOutput=6  RepetitionCount=0  Input0Tiling=mtxA_w(1)  Input1Tiling=mtxA_w(2)  Input2Tiling=mtxA_w(3)  Input3Tiling=[]  Input4Tiling=[]  Input5Tiling=[]  Output0Tiling=mtxA_r(1)  Output1Tiling=mtxA_r(2)  Output2Tiling=mtxA_r(3)  Output3Tiling=mtxA_r(4)  Output4Tiling=mtxA_r(5)  Output5Tiling=mtxA_r(6)  InBuffDims={128, 384}|{128, 384}|{128, 384}  InTilingDims={128, 128}|{128, 128}|{128, 128}  InOffsets={0, 0}|{0, 128}|{0, 256}  InTileTraveseDims={}|{}|{}  InTileTraveseStrides={}|{}|{}  InTileTraveseWraps={}|{}|{}  InPacketPortIDs={}|{}|{}  InRepetitions={}|{}|{}  InPhases={}|{}|{}  InBoundaryDims={}|{}|{}  OutBuffDims={128, 384}|{128, 384}|{128, 384}|{128, 384}|{128, 384}|{128, 384}  OutTilingDims={128, 64}|{128, 64}|{128, 64}|{128, 64}|{128, 64}|{128, 64}  OutOffsets={0, 0}|{0, 64}|{0, 128}|{0, 192}|{0, 256}|{0, 320}  OutTileTraveseDims={}|{}|{}|{}|{}|{}  OutTileTraveseStrides={}|{}|{}|{}|{}|{}  OutTileTraveseWraps={}|{}|{}|{}|{}|{}  OutPacketPortIDs={}|{}|{}|{}|{}|{}  OutRepetitions={}|{}|{}|{}|{}|{}  OutPhases={}|{}|{}|{}|{}|{}  OutBoundaryDims={}|{}|{}|{}|{}|{}  BufferDimStr={256, 384}  blockJsonConstraints=[]  deprecateConstraints=0
  mtxB : aieBasic/Shared Buffer  DataType=bfloat16  NumBuffer=1  BufferDim=[COL,ROW]  NumInput=6  NumOutput=3  RepetitionCount=0  Input0Tiling=mtxB_w(1)  Input1Tiling=mtxB_w(2)  Input2Tiling=mtxB_w(3)  Input3Tiling=mtxB_w(4)  Input4Tiling=mtxB_w(5)  Input5Tiling=mtxB_w(6)  Output0Tiling=mtxB_r(1)  Output1Tiling=mtxB_r(2)  Output2Tiling=mtxB_r(3)  Output3Tiling=struct('buffer_dimension', [256,384], 'tiling_dimension', [256,64], 'offset', [0,64*3])  Output4Tiling=struct('buffer_dimension', [256,384], 'tiling_dimension', [256,64], 'offset', [0,64*4])  Output5Tiling=struct('buffer_dimension', [256,384], 'tiling_dimension', [256,64], 'offset', [0,64*5])  InBuffDims={128, 384}|{128, 384}|{128, 384}|{128, 384}|{128, 384}|{128, 384}  InTilingDims={128, 64}|{128, 64}|{128, 64}|{128, 64}|{128, 64}|{128, 64}  InOffsets={0, 0}|{0, 64}|{0, 128}|{0, 192}|{0, 256}|{0, 320}  InTileTraveseDims={}|{}|{}|{}|{}|{}  InTileTraveseStrides={}|{}|{}|{}|{}|{}  InTileTraveseWraps={}|{}|{}|{}|{}|{}  InPacketPortIDs={}|{}|{}|{}|{}|{}  InRepetitions={}|{}|{}|{}|{}|{}  InPhases={}|{}|{}|{}|{}|{}  InBoundaryDims={}|{}|{}|{}|{}|{}  OutBuffDims={128, 384}|{128, 384}|{128, 384}  OutTilingDims={128, 128}|{128, 128}|{128, 128}  OutOffsets={0, 0}|{0, 128}|{0, 256}  OutTileTraveseDims={}|{}|{}  OutTileTraveseStrides={}|{}|{}  OutTileTraveseWraps={}|{}|{}  OutPacketPortIDs={}|{}|{}  OutRepetitions={}|{}|{}  OutPhases={}|{}|{}  OutBoundaryDims={}|{}|{}  BufferDimStr={256, 384}  blockJsonConstraints=[]  deprecateConstraints=0
  Out1 : Outport
  Out2 : Outport  Port=2
  Out3 : Outport  Port=3
  wires:
  PLIO5/1 -> Out3/1
  mean_dev_norm_middle3/2 -> mean_dev_norm_last/2
  PLIO2/1 -> mtxA/3
  mean_dev_norm_middle2/2 -> mean_dev_norm_middle3/3
  mtxB/3 -> PLIO5/1
  In1/1 -> PLIO/1
  PLIO3/1 -> Out1/1
  mean_dev_norm_middle/1 -> mtxB/2
  mean_dev_norm_last/1 -> mtxB/6
  PLIO4/1 -> Out2/1
  mean_dev_norm_middle1/1 -> mtxB/3
  mtxB/2 -> PLIO4/1
  mean_dev_norm_middle3/1 -> mtxB/5
  mtxB/1 -> PLIO3/1
  PLIO/1 -> mtxA/1
  PLIO1/1 -> mtxA/2
  mean_dev_norm_middle2/1 -> mtxB/4
  mean_dev_norm_middle1/2 -> mean_dev_norm_middle2/3
  mtxA/1 -> mean_dev_norm_first/1
  mean_dev_norm_first/2 -> mean_dev_norm_middle/3
  mtxA/3 -> mean_dev_norm_middle1/1
  mtxA/4 -> mean_dev_norm_middle2/1
  mtxA/5 -> mean_dev_norm_middle3/1
  mtxA/6 -> mean_dev_norm_last/1
  mean_dev_norm_last/2 -> Convert From Bfloat16/1
  MATLAB System/1 -> Convert To Bfloat1/1
  Convert To Bfloat1/1 -> mean_dev_norm_first/2, mean_dev_norm_middle/2, mean_dev_norm_middle1/2, mean_dev_norm_middle2/2, mean_dev_norm_middle3/2
  Convert From Bfloat16/1 -> MATLAB System/1
  In2/1 -> PLIO1/1
  In3/1 -> PLIO2/1
  mean_dev_norm_middle/2 -> mean_dev_norm_middle1/3
  mtxA/2 -> mean_dev_norm_middle/1
  mean_dev_norm_first/1 -> mtxB/1
